simulink library "RWS_1W_PDcontroller"  (R2018a)
settings: Solver=ode45  StartTime=0.0  StopTime=10.0  RelTol=1e-3  EnableMultiTasking=on
undefined symbols (not defined in the file): ConfParam
libraries: Qerror x1
settings Model: Creator=Hp  LastModifiedBy=Cédric
settings DataIOCC: LimitDataPoints=on  SaveFormat=Array
settings OptimizationCC: LifeSpan=inf
settings DebuggingCC: SolverPrmCheckMsg=warning  SFUnexpectedBacktrackingDiag=warning  SFNoUnconditionalDefaultTransitionDiag=warning  SFExecutionAtInitializationDiag=none
settings HardwareCC: ProdBitPerPointer=32  ProdBitPerSizeT=32  ProdBitPerPtrDiffT=32  ProdLargestAtomicFloat=None  ProdIntDivRoundTo=Undefined  ProdEndianess=Unspecified  ProdWordSize=32  ProdHWDeviceType=32-bit Generic
settings ModelReferenceCC: PropagateSignalLabelsOutOfModel=off
settings CodeAppCC: StateflowObjectComments=on
settings GRTTargetCC: TargetLangStandard=C89/C90 (ANSI)  GeneratePreprocessorConditionals=Disable all
settings ConfigComp: CovMetricSettings=dw  CovHtmlReporting=on  CovSaveCumulativeToWorkspaceVar=on  CovSaveSingleToWorkspaceVar=on  CovExternalEMLEnable=off  CovSFcnEnable=off

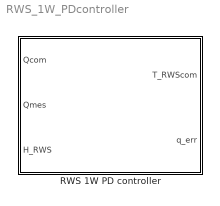
== system RWS_1W_PDcontroller ==
  RWS 1W PD controller : Subsystem

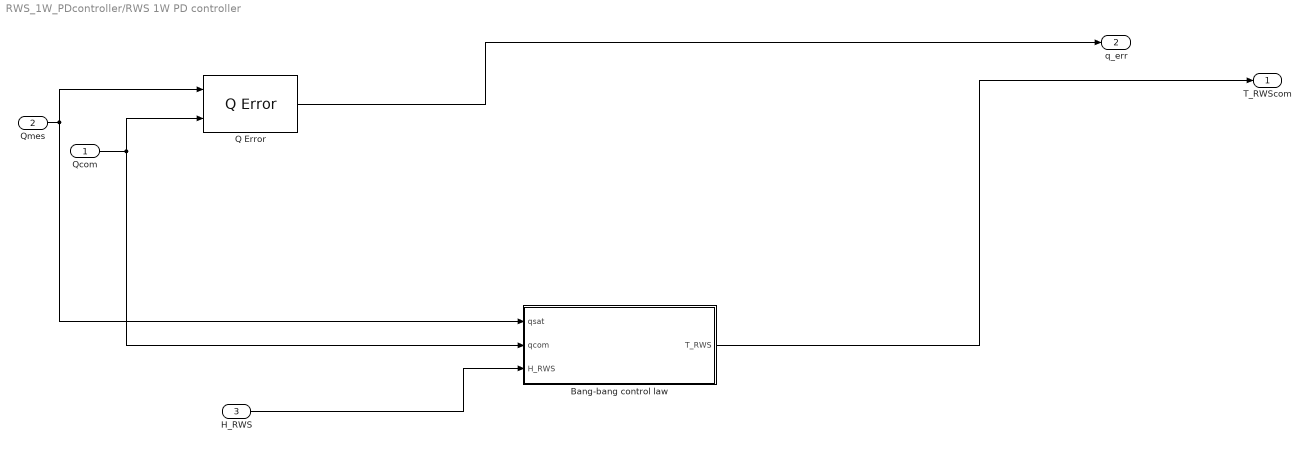
== system RWS_1W_PDcontroller/RWS 1W PD controller ==
  Qcom : Inport
  Qmes : Inport  Port=2
  H_RWS : Inport  Port=3
  Bang-bang control law : Subsystem
  Q Error : Qerror/Q Error
  T_RWScom : Outport
  q_err : Outport  Port=2
  wires:
  Bang-bang control law/1(T_RWS) -> T_RWScom/1
  H_RWS/1 -> Bang-bang control law/3(H_RWS)
  Qcom/1 -> Q Error/2, Bang-bang control law/2(qcom)
  Qmes/1 -> Q Error/1, Bang-bang control law/1(qsat)
  Q Error/1 -> q_err/1

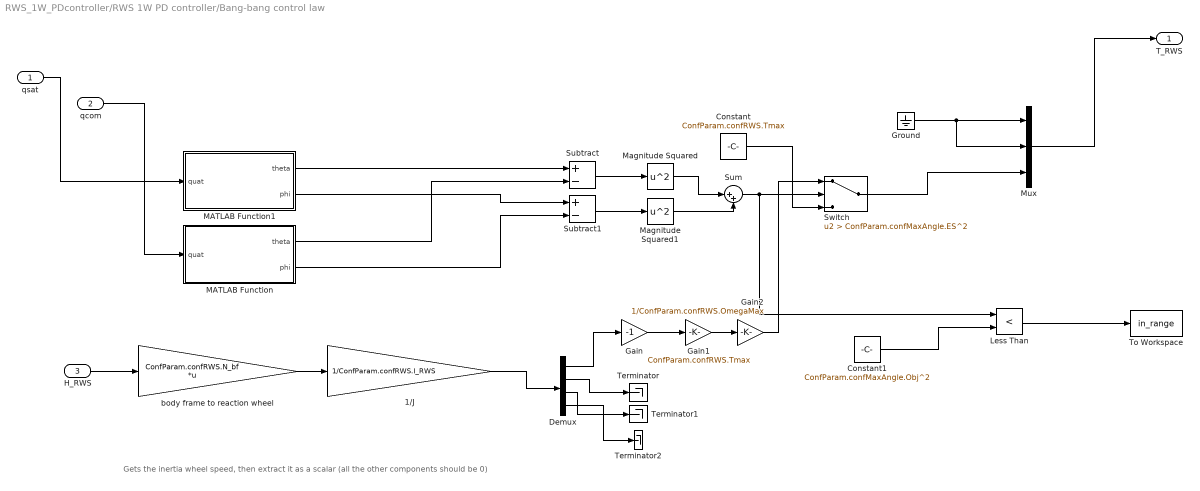
== system RWS_1W_PDcontroller/RWS 1W PD controller/Bang-bang control law ==
  note: Gets the inertia wheel speed, then extract it as a scalar (all the other components should be 0)
  qsat : Inport
  qcom : Inport  Port=2
  H_RWS : Inport  Port=3
  1/J : Gain  Gain=1/ConfParam.confRWS.I_RWS
  Constant : Constant  Value=ConfParam.confRWS.Tmax
  Constant1 : Constant  Value=ConfParam.confMaxAngle.Obj^2
  Demux : Demux
  Gain : Gain  Gain=-1
  Gain1 : Gain  Gain=ConfParam.confRWS.Tmax
  Gain2 : Gain  Gain=1/ConfParam.confRWS.OmegaMax
  Ground : Ground
  Less Than : RelationalOperator  Operator=<  OutDataTypeStr=boolean  RndMeth=Simplest
  MATLAB Function : MATLAB Function  TreatAsAtomicUnit=on
  MATLAB Function1 : MATLAB Function  TreatAsAtomicUnit=on
  Magnitude Squared : Math  Operator=square  SaturateOnIntegerOverflow=on
  Magnitude Squared1 : Math  Operator=square  SaturateOnIntegerOverflow=on
  Mux : Mux  Inputs=3
  Subtract : Sum  Inputs=+-
  Subtract1 : Sum  Inputs=+-
  Sum : Sum  Inputs=|++
  Switch : Switch  Criteria=u2 > Threshold  Threshold=ConfParam.confMaxAngle.ES^2
  Terminator : Terminator
  Terminator1 : Terminator
  Terminator2 : Terminator
  To Workspace : ToWorkspace  VariableName=in_range  SampleTime=-1
  body frame to reaction wheel : Gain  Gain=ConfParam.confRWS.N_bf  Multiplication=Matrix(K*u)
  T_RWS : Outport
  wires:
  Gain1/1 -> Gain2/1
  Less Than/1 -> To Workspace/1
  Gain/1 -> Gain1/1
  Constant1/1 -> Less Than/2
  1/J/1 -> Demux/1
  Mux/1 -> T_RWS/1
  body frame to reaction wheel/1 -> 1/J/1
  MATLAB Function1/1(theta) -> Subtract/1
  Sum/1 -> Less Than/1, Switch/2
  Subtract/1 -> Magnitude Squared/1
  Magnitude Squared/1 -> Sum/1
  MATLAB Function1/2(phi) -> Subtract1/1
  Subtract1/1 -> Magnitude Squared1/1
  MATLAB Function/1(theta) -> Subtract/2
  qcom/1 -> MATLAB Function/1(quat)
  Magnitude Squared1/1 -> Sum/2
  Demux/2 -> Terminator/1
  H_RWS/1 -> body frame to reaction wheel/1
  Demux/3 -> Terminator1/1
  MATLAB Function/2(phi) -> Subtract1/2
  qsat/1 -> MATLAB Function1/1(quat)
  Demux/4 -> Terminator2/1
  Demux/1 -> Gain/1
  Switch/1 -> Mux/3
  Ground/1 -> Mux/2, Mux/1
  Constant/1 -> Switch/3
  Gain2/1 -> Switch/1

== matlab function RWS_1W_PDcontroller/RWS 1W PD controller/Bang-bang control law/MATLAB Function1 ==
  data: quat input; theta output; phi output
function [theta, phi] = extract_sph_angles(quat)

%%% extracts theta and phi from quaternion qsat
%%% here we consider the angles for the z-axis (0 0 1)
%%% but it can be changed to any other axis if necessary.

q0 = quat(1);
q1 = quat(2);
q2 = quat(3);
q3 = quat(4);
P = [2*(q0^2 + q1^2)-1 2*(q1*q2 - q0*q3) 2*(q1*q3 + q2*q0);
     2*(q1*q2 + q0*q3) 2*(q0^2 + q2^2)-1 2*(q2*q3 - q1*q0);
     2*(q1*q3 - q2*q0) 2*(q2*q3 + q1*q0) 2*(q0^2 + q3^2)-1];
prod = P*[0; 0; 1];
x = prod(1);
y = prod(2);
z = prod(3);
[phi, theta, r] = cart2sph(x, y, z);

== matlab function RWS_1W_PDcontroller/RWS 1W PD controller/Bang-bang control law/MATLAB Function ==
  data: quat input; theta output; phi output
function [theta, phi] = extract_sph_angles(quat)

%%% extracts theta and phi from quaternion qsat
%%% here we consider the angles for the z-axis (0 0 1)
%%% but it can be changed to any other axis if necessary.

q0 = quat(1);
q1 = quat(2);
q2 = quat(3);
q3 = quat(4);
P = [2*(q0^2 + q1^2)-1 2*(q1*q2 - q0*q3) 2*(q1*q3 + q2*q0);
     2*(q1*q2 + q0*q3) 2*(q0^2 + q2^2)-1 2*(q2*q3 - q1*q0);
     2*(q1*q3 - q2*q0) 2*(q2*q3 + q1*q0) 2*(q0^2 + q3^2)-1];
prod = P*[0; 0; 1];
x = prod(1);
y = prod(2);
z = prod(3);
[phi, theta, r] = cart2sph(x, y, z);
